simulink model "Physical_Architecture"  (R2025b)
settings: Solver=VariableStepAuto  StartTime=0.0  StopTime=10.0  RelTol=1e-3
settings Model: Creator=shrig  LastModifiedBy=shrig

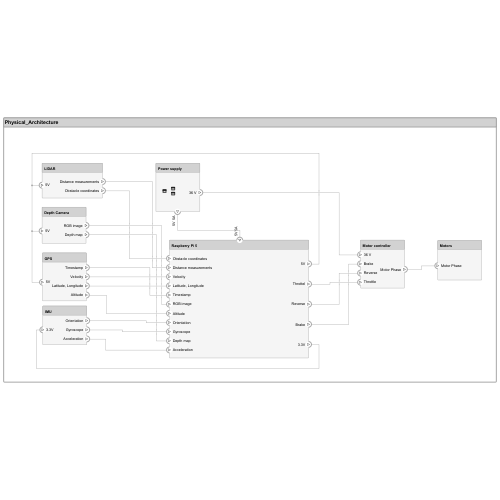
[thumbnail: Simulink's stored preview of the top-level diagram]
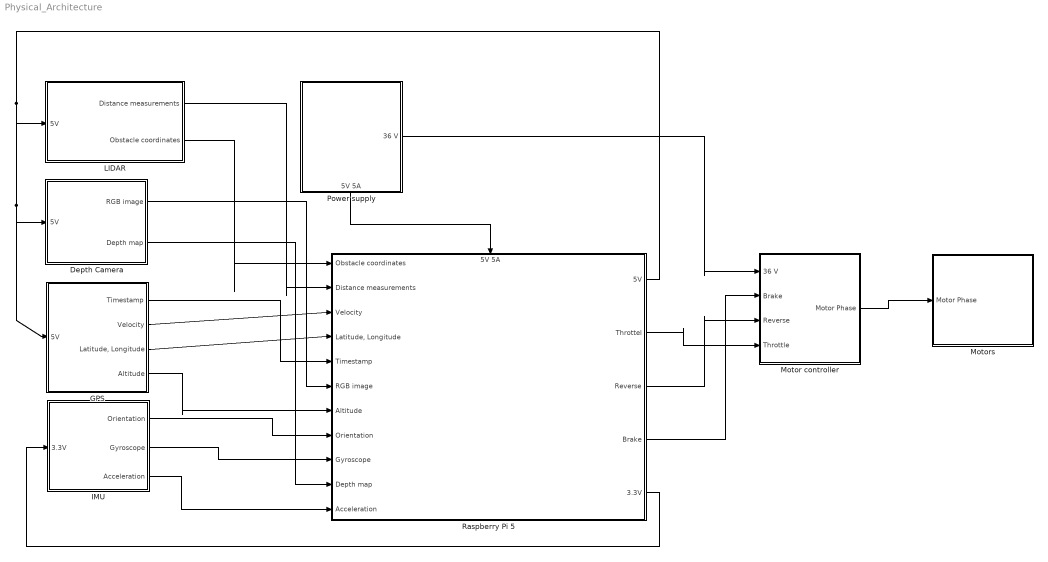
== system Physical_Architecture ==
  Depth Camera : Subsystem
      settings: PortSchema="{\"entries\":[{\"content\":{\"headerSize\":26,\"margin\":15,\"minimumSpacing\":25,\"sides\":[{\"content\":{\"connectorIds\":[\"In1\"]},\"type\":\"ConnectorPlacement.EquallySpacedRectSide\",\"uuid\":\"9d85ba2d-7d52-4590-a2a8-50caab8edece\"},{\"content\":{\"connectorIds\":[\"Out1\",\"Out2\"],\"side\":\"RIGHT\"},\"type\":\"ConnectorPlacement.EquallySpacedRectSide\",\"uuid\":\"20a8f066-7868-465b-8d14-5c46bf5e912a\"},{\"content\":{\"side\":\"TOP\"},\"type\":\"ConnectorPlacement.EquallySpacedRectSide\",\"uuid\":\"e28b85aa-6bfa-4f90-b1ed-762b348e72e7\"}]},\"type\":\"ConnectorPlacement.EquallySpacedConnector\",\"uuid\":\"b4aeeca3-9a94-45ab-bd39-d35b188e9431\"}],\"packageUris\":[\"http://schema.mathworks.com/mf0/Connector/R2020b\"],\"version\":\"1.0\"}"
  GPS : Subsystem
      settings: PortSchema="{\"entries\":[{\"content\":{\"headerSize\":26,\"margin\":15,\"minimumSpacing\":25,\"sides\":[{\"content\":{\"connectorIds\":[\"In1\"]},\"type\":\"ConnectorPlacement.EquallySpacedRectSide\",\"uuid\":\"9d85ba2d-7d52-4590-a2a8-50caab8edece\"},{\"content\":{\"connectorIds\":[\"Out1\",\"Out2\",\"Out3\",\"Out4\"],\"side\":\"RIGHT\"},\"type\":\"ConnectorPlacement.EquallySpacedRectSide\",\"uuid\":\"20a8f066-7868-465b-8d14-5c46bf5e912a\"},{\"content\":{\"side\":\"TOP\"},\"type\":\"ConnectorPlacement.EquallySpacedRectSide\",\"uuid\":\"e28b85aa-6bfa-4f90-b1ed-762b348e72e7\"}]},\"type\":\"ConnectorPlacement.EquallySpacedConnector\",\"uuid\":\"b4aeeca3-9a94-45ab-bd39-d35b188e9431\"}],\"packageUris\":[\"http://schema.mathworks.com/mf0/Connector/R2020b\"],\"version\":\"1.0\"}"
  IMU : Subsystem
      settings: PortSchema="{\"entries\":[{\"content\":{\"headerSize\":26,\"margin\":15,\"minimumSpacing\":25,\"sides\":[{\"content\":{\"connectorIds\":[\"In1\"]},\"type\":\"ConnectorPlacement.EquallySpacedRectSide\",\"uuid\":\"9d85ba2d-7d52-4590-a2a8-50caab8edece\"},{\"content\":{\"connectorIds\":[\"Out1\",\"Out2\",\"Out3\"],\"side\":\"RIGHT\"},\"type\":\"ConnectorPlacement.EquallySpacedRectSide\",\"uuid\":\"20a8f066-7868-465b-8d14-5c46bf5e912a\"},{\"content\":{\"side\":\"TOP\"},\"type\":\"ConnectorPlacement.EquallySpacedRectSide\",\"uuid\":\"e28b85aa-6bfa-4f90-b1ed-762b348e72e7\"}]},\"type\":\"ConnectorPlacement.EquallySpacedConnector\",\"uuid\":\"b4aeeca3-9a94-45ab-bd39-d35b188e9431\"}],\"packageUris\":[\"http://schema.mathworks.com/mf0/Connector/R2020b\"],\"version\":\"1.0\"}"
  LIDAR : Subsystem
      settings: PortSchema="{\"entries\":[{\"content\":{\"headerSize\":26,\"margin\":15,\"minimumSpacing\":25,\"sides\":[{\"content\":{\"connectorIds\":[\"In1\"]},\"type\":\"ConnectorPlacement.EquallySpacedRectSide\",\"uuid\":\"9d85ba2d-7d52-4590-a2a8-50caab8edece\"},{\"content\":{\"connectorIds\":[\"Out2\",\"Out1\"],\"side\":\"RIGHT\"},\"type\":\"ConnectorPlacement.EquallySpacedRectSide\",\"uuid\":\"20a8f066-7868-465b-8d14-5c46bf5e912a\"},{\"content\":{\"side\":\"TOP\"},\"type\":\"ConnectorPlacement.EquallySpacedRectSide\",\"uuid\":\"e28b85aa-6bfa-4f90-b1ed-762b348e72e7\"}]},\"type\":\"ConnectorPlacement.EquallySpacedConnector\",\"uuid\":\"b4aeeca3-9a94-45ab-bd39-d35b188e9431\"}],\"packageUris\":[\"http://schema.mathworks.com/mf0/Connector/R2020b\"],\"version\":\"1.0\"}"
  Motor controller : Subsystem
      settings: PortSchema="{\"entries\":[{\"content\":{\"headerSize\":26,\"margin\":15,\"minimumSpacing\":25,\"sides\":[{\"content\":{\"connectorIds\":[\"In1\",\"In2\",\"In3\",\"In4\"]},\"type\":\"ConnectorPlacement.EquallySpacedRectSide\",\"uuid\":\"9d85ba2d-7d52-4590-a2a8-50caab8edece\"},{\"content\":{\"connectorIds\":[\"Out1\"],\"side\":\"RIGHT\"},\"type\":\"ConnectorPlacement.EquallySpacedRectSide\",\"uuid\":\"20a8f066-7868-465b-8d14-5c46bf5e912a\"},{\"content\":{\"side\":\"TOP\"},\"type\":\"ConnectorPlacement.EquallySpacedRectSide\",\"uuid\":\"e28b85aa-6bfa-4f90-b1ed-762b348e72e7\"}]},\"type\":\"ConnectorPlacement.EquallySpacedConnector\",\"uuid\":\"b4aeeca3-9a94-45ab-bd39-d35b188e9431\"}],\"packageUris\":[\"http://schema.mathworks.com/mf0/Connector/R2020b\"],\"version\":\"1.0\"}"
  "Motors " : Subsystem
      settings: PortSchema="{\"entries\":[{\"content\":{\"headerSize\":26,\"margin\":15,\"minimumSpacing\":25,\"sides\":[{\"content\":{\"connectorIds\":[\"In1\"]},\"type\":\"ConnectorPlacement.EquallySpacedRectSide\",\"uuid\":\"9d85ba2d-7d52-4590-a2a8-50caab8edece\"},{\"content\":{\"side\":\"RIGHT\"},\"type\":\"ConnectorPlacement.EquallySpacedRectSide\",\"uuid\":\"20a8f066-7868-465b-8d14-5c46bf5e912a\"},{\"content\":{\"side\":\"TOP\"},\"type\":\"ConnectorPlacement.EquallySpacedRectSide\",\"uuid\":\"e28b85aa-6bfa-4f90-b1ed-762b348e72e7\"}]},\"type\":\"ConnectorPlacement.EquallySpacedConnector\",\"uuid\":\"b4aeeca3-9a94-45ab-bd39-d35b188e9431\"}],\"packageUris\":[\"http://schema.mathworks.com/mf0/Connector/R2020b\"],\"version\":\"1.0\"}"
  Power supply : Subsystem
      settings: PortSchema="{\"entries\":[{\"content\":{\"headerSize\":26,\"margin\":15,\"minimumSpacing\":25,\"sides\":[{\"content\":{},\"type\":\"ConnectorPlacement.EquallySpacedRectSide\",\"uuid\":\"9d85ba2d-7d52-4590-a2a8-50caab8edece\"},{\"content\":{\"connectorIds\":[\"Out1\"],\"side\":\"RIGHT\"},\"type\":\"ConnectorPlacement.EquallySpacedRectSide\",\"uuid\":\"20a8f066-7868-465b-8d14-5c46bf5e912a\"},{\"content\":{\"side\":\"TOP\"},\"type\":\"ConnectorPlacement.EquallySpacedRectSide\",\"uuid\":\"e28b85aa-6bfa-4f90-b1ed-762b348e72e7\"},{\"content\":{\"connectorIds\":[\"Out2\"],\"side\":\"BOTTOM\"},\"type\":\"ConnectorPlacement.EquallySpacedRectSide\",\"uuid\":\"bd4d5535-b116-44ab-93c6-78de3977892e\"}]},\"type\":\"ConnectorPlacement.EquallySpacedConnector\",\"uuid\":\"b4aeeca3-9a94-45ab-bd39-d35b188e9431\"}],\"packageUris\":[\"http://schema.mathworks.com/mf0/Connector/R2020b\"],\"version\":\"1.0\"}"
  Raspberry Pi 5 : Subsystem
      settings: PortSchema="{\"entries\":[{\"content\":{\"headerSize\":26,\"margin\":15,\"minimumSpacing\":25,\"sides\":[{\"content\":{\"connectorIds\":[\"In1\",\"In2\",\"In3\",\"In4\",\"In5\",\"In6\",\"In7\",\"In8\",\"In9\",\"In10\",\"In12\"]},\"type\":\"ConnectorPlacement.EquallySpacedRectSide\",\"uuid\":\"9d85ba2d-7d52-4590-a2a8-50caab8edece\"},{\"content\":{\"connectorIds\":[\"Out1\",\"Out2\",\"Out3\",\"Out4\",\"Out5\"],\"side\":\"RIGHT\"},\"type\":\"ConnectorPlacement.EquallySpacedRectSide\",\"uuid\":\"20a8f066-7868-465b-8d14-5c46bf5e912a\"},{\"content\":{\"connectorIds\":[\"In11\"],\"side\":\"TOP\"},\"type\":\"ConnectorPlacement.EquallySpacedRectSide\",\"uuid\":\"e28b85aa-6bfa-4f90-b1ed-762b348e72e7\"}]},\"type\":\"ConnectorPlacement.EquallySpacedConnector\",\"uuid\":\"b4aeeca3-9a94-45ab-bd39-d35b188e9431\"}],\"packageUris\":[\"http://schema.mathworks.com/mf0/Connector/R2020b\"],\"version\":\"1.0\"}"
  wires:
  IMU/3(Acceleration) -> Raspberry Pi 5/12(Acceleration)
  Power supply/2(5V 5A) -> Raspberry Pi 5/11(5V 5A)
  Depth Camera/2(Depth map) -> Raspberry Pi 5/10(Depth map)
  LIDAR/2(Distance measurements) -> Raspberry Pi 5/2(Distance measurements)
  GPS/4(Altitude) -> Raspberry Pi 5/7(Altitude)
  Power supply/1(36 V) -> Motor controller/1(36 V)
  Raspberry Pi 5/4(Brake) -> Motor controller/2(Brake)
  Raspberry Pi 5/1(5V) -> GPS/1(5V), Depth Camera/1(5V), LIDAR/1(5V)
  Raspberry Pi 5/5(3.3V) -> IMU/1(3.3V)
  Depth Camera/1(RGB image) -> Raspberry Pi 5/6(RGB image)
  LIDAR/1(Obstacle coordinates) -> Raspberry Pi 5/1(Obstacle coordinates)
  GPS/1(Timestamp) -> Raspberry Pi 5/5(Timestamp)
  GPS/2(Velocity) -> Raspberry Pi 5/3(Velocity)
  GPS/3("Latitude, Longitude") -> Raspberry Pi 5/4("Latitude, Longitude")
  IMU/1(Orientation) -> Raspberry Pi 5/8(Orientation)
  IMU/2(Gyroscope) -> Raspberry Pi 5/9(Gyroscope)
  Motor controller/1(Motor Phase) -> "Motors "/1(Motor Phase)
  Raspberry Pi 5/2(Throttel) -> Motor controller/4(Throttle)
  Raspberry Pi 5/3(Reverse) -> Motor controller/3(Reverse)

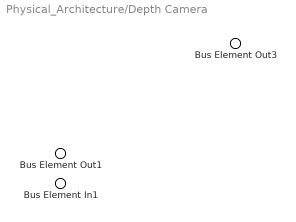
== system Physical_Architecture/Depth Camera ==
  Bus Element In1 : Inport  PortName=5V
  Bus Element Out3 : Outport  PortName=RGB image
  Bus Element Out1 : Outport  Port=2  PortName=Depth map

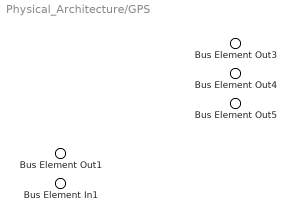
== system Physical_Architecture/GPS ==
  Bus Element In1 : Inport  PortName=5V
  Bus Element Out5 : Outport  PortName=Timestamp
  Bus Element Out4 : Outport  Port=2  PortName=Velocity
  Bus Element Out3 : Outport  Port=3  PortName=Latitude, Longitude
  Bus Element Out1 : Outport  Port=4  PortName=Altitude

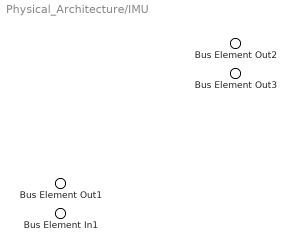
== system Physical_Architecture/IMU ==
  Bus Element In1 : Inport  PortName=3.3V
  Bus Element Out3 : Outport  PortName=Orientation
  Bus Element Out2 : Outport  Port=2  PortName=Gyroscope
  Bus Element Out1 : Outport  Port=3  PortName=Acceleration

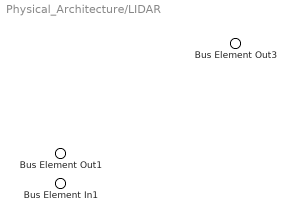
== system Physical_Architecture/LIDAR ==
  Bus Element In1 : Inport  PortName=5V
  Bus Element Out3 : Outport  PortName=Obstacle coordinates
  Bus Element Out1 : Outport  Port=2  PortName=Distance measurements

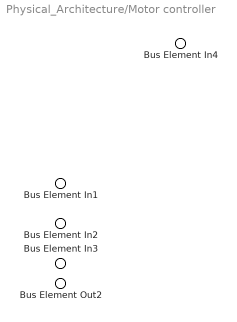
== system Physical_Architecture/Motor controller ==
  Bus Element In1 : Inport  PortName=36 V
  Bus Element In2 : Inport  Port=2  PortName=Brake
  Bus Element In4 : Inport  Port=3  PortName=Reverse
  Bus Element In3 : Inport  Port=4  PortName=Throttle
  Bus Element Out2 : Outport  PortName=Motor Phase

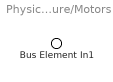
== system Physical_Architecture/Motors  ==
  Bus Element In1 : Inport  PortName=Motor Phase

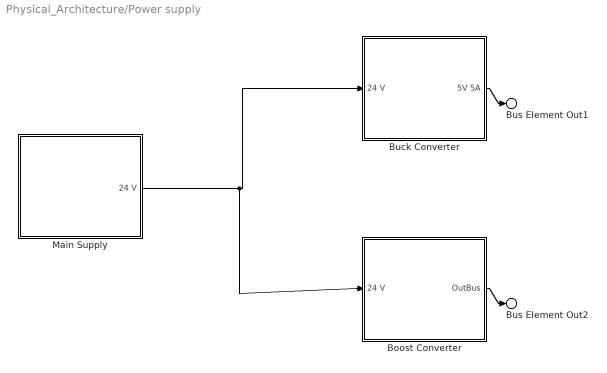
== system Physical_Architecture/Power supply ==
  Boost Converter : Subsystem
      settings: PortSchema="{\"entries\":[{\"content\":{\"headerSize\":26,\"margin\":15,\"minimumSpacing\":25,\"sides\":[{\"content\":{\"connectorIds\":[\"In1\"]},\"type\":\"ConnectorPlacement.EquallySpacedRectSide\",\"uuid\":\"9d85ba2d-7d52-4590-a2a8-50caab8edece\"},{\"content\":{\"connectorIds\":[\"Out1\"],\"side\":\"RIGHT\"},\"type\":\"ConnectorPlacement.EquallySpacedRectSide\",\"uuid\":\"20a8f066-7868-465b-8d14-5c46bf5e912a\"},{\"content\":{\"side\":\"TOP\"},\"type\":\"ConnectorPlacement.EquallySpacedRectSide\",\"uuid\":\"e28b85aa-6bfa-4f90-b1ed-762b348e72e7\"}]},\"type\":\"ConnectorPlacement.EquallySpacedConnector\",\"uuid\":\"b4aeeca3-9a94-45ab-bd39-d35b188e9431\"}],\"packageUris\":[\"http://schema.mathworks.com/mf0/Connector/R2020b\"],\"version\":\"1.0\"}"
  Buck Converter : Subsystem
      settings: PortSchema="{\"entries\":[{\"content\":{\"headerSize\":26,\"margin\":15,\"minimumSpacing\":25,\"sides\":[{\"content\":{\"connectorIds\":[\"In1\"]},\"type\":\"ConnectorPlacement.EquallySpacedRectSide\",\"uuid\":\"9d85ba2d-7d52-4590-a2a8-50caab8edece\"},{\"content\":{\"connectorIds\":[\"Out1\"],\"side\":\"RIGHT\"},\"type\":\"ConnectorPlacement.EquallySpacedRectSide\",\"uuid\":\"20a8f066-7868-465b-8d14-5c46bf5e912a\"},{\"content\":{\"side\":\"TOP\"},\"type\":\"ConnectorPlacement.EquallySpacedRectSide\",\"uuid\":\"e28b85aa-6bfa-4f90-b1ed-762b348e72e7\"}]},\"type\":\"ConnectorPlacement.EquallySpacedConnector\",\"uuid\":\"b4aeeca3-9a94-45ab-bd39-d35b188e9431\"}],\"packageUris\":[\"http://schema.mathworks.com/mf0/Connector/R2020b\"],\"version\":\"1.0\"}"
  "Main Supply " : Subsystem
      settings: PortSchema="{\"entries\":[{\"content\":{\"headerSize\":26,\"margin\":15,\"minimumSpacing\":25,\"sides\":[{\"content\":{},\"type\":\"ConnectorPlacement.EquallySpacedRectSide\",\"uuid\":\"9d85ba2d-7d52-4590-a2a8-50caab8edece\"},{\"content\":{\"connectorIds\":[\"Out1\"],\"side\":\"RIGHT\"},\"type\":\"ConnectorPlacement.EquallySpacedRectSide\",\"uuid\":\"20a8f066-7868-465b-8d14-5c46bf5e912a\"},{\"content\":{\"side\":\"TOP\"},\"type\":\"ConnectorPlacement.EquallySpacedRectSide\",\"uuid\":\"e28b85aa-6bfa-4f90-b1ed-762b348e72e7\"}]},\"type\":\"ConnectorPlacement.EquallySpacedConnector\",\"uuid\":\"b4aeeca3-9a94-45ab-bd39-d35b188e9431\"}],\"packageUris\":[\"http://schema.mathworks.com/mf0/Connector/R2020b\"],\"version\":\"1.0\"}"
  Bus Element Out2 : Outport  PortName=36 V
  Bus Element Out1 : Outport  Port=2  PortName=5V 5A
  wires:
  "Main Supply "/1(24 V) -> Boost Converter/1(24 V), Buck Converter/1(24 V)
  Buck Converter/1(5V 5A) -> Bus Element Out1/1
  Boost Converter/1(OutBus) -> Bus Element Out2/1

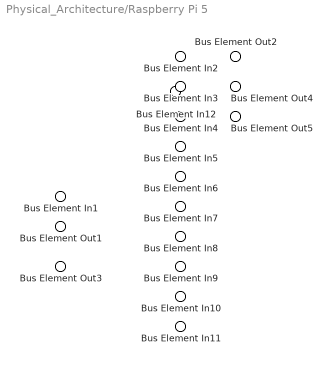
== system Physical_Architecture/Raspberry Pi 5 ==
  Bus Element In7 : Inport  PortName=Obstacle coordinates
  Bus Element In4 : Inport  Port=2  PortName=Distance measurements
  Bus Element In9 : Inport  Port=3  PortName=Velocity
  Bus Element In10 : Inport  Port=4  PortName=Latitude, Longitude
  Bus Element In8 : Inport  Port=5  PortName=Timestamp
  Bus Element In6 : Inport  Port=6  PortName=RGB image
  Bus Element In5 : Inport  Port=7  PortName=Altitude
  Bus Element In11 : Inport  Port=8  PortName=Orientation
  Bus Element In12 : Inport  Port=9  PortName=Gyroscope
  Bus Element In3 : Inport  Port=10  PortName=Depth map
  Bus Element In2 : Inport  Port=11  PortName=5V 5A
  Bus Element In1 : Inport  Port=12  PortName=Acceleration
  Bus Element Out2 : Outport  PortName=5V
  Bus Element Out4 : Outport  Port=2  PortName=Throttel
  Bus Element Out5 : Outport  Port=3  PortName=Reverse
  Bus Element Out1 : Outport  Port=4  PortName=Brake
  Bus Element Out3 : Outport  Port=5  PortName=3.3V

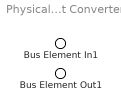
== system Physical_Architecture/Power supply/Boost Converter ==
  Bus Element In1 : Inport  PortName=24 V
  Bus Element Out1 : Outport  PortName=OutBus

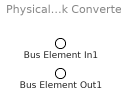
== system Physical_Architecture/Power supply/Buck Converter ==
  Bus Element In1 : Inport  PortName=24 V
  Bus Element Out1 : Outport  PortName=5V 5A

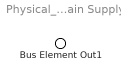
== system Physical_Architecture/Power supply/Main Supply  ==
  Bus Element Out1 : Outport  PortName=24 V
